simulink model "controller_test_lqg"  (R2015a)
settings: Solver=FixedStepDiscrete  StartTime=0.0  StopTime=40  FixedStep=0.02  RelTol=1e-3
values from neighbouring files (symbols this model uses):
  A = [2.32106176877 1 0 0 0 0 0 -0.677256428753 0 1 0 0 ... (49 elements, 7x7)]    [identified_sys_model.mat]
  B = [1 0 0 0 0 0 0]    [identified_sys_model.mat]
  C = [-0.0947664146756 0.174494212895 0 0 0 0 0]    [identified_sys_model.mat]
  M = iddata(yf2,u2detrended)    [model_identification_tests.m]
  Nbar = Nu+K*Nx    [controller_test.m]
undefined symbols (not defined in the file or in its folder): K
settings Model: ExtModeTrigDuration=200000  Creator=alunos  LastModifiedBy=jmgri
settings DataIOCC: LimitDataPoints=off
settings HardwareCC: ProdBitPerPointer=64  ProdLargestAtomicFloat=Float  ProdIntDivRoundTo=Zero  ProdEndianess=LittleEndian  ProdHWDeviceType=Specified  TargetIntDivRoundTo=Zero  TargetEndianess=LittleEndian  TargetHWDeviceType=Intel->x86/Pentium
settings RTWCC: SystemTargetFile=rtwin.tlc  TemplateMakefile=rtwin.tmf  Description=Simulink Desktop Real-Time  RTWCompilerOptimization=on
settings CodeAppCC: MaxIdLength=95
settings RTWinTargetCC: TargetPreCompLibLocation=C:\Program Files\MATLAB\R2017a\toolbox\sldrt\lib\win64  GeneratePreprocessorConditionals=Use local settings  ExtModeMexFile=sldrtext

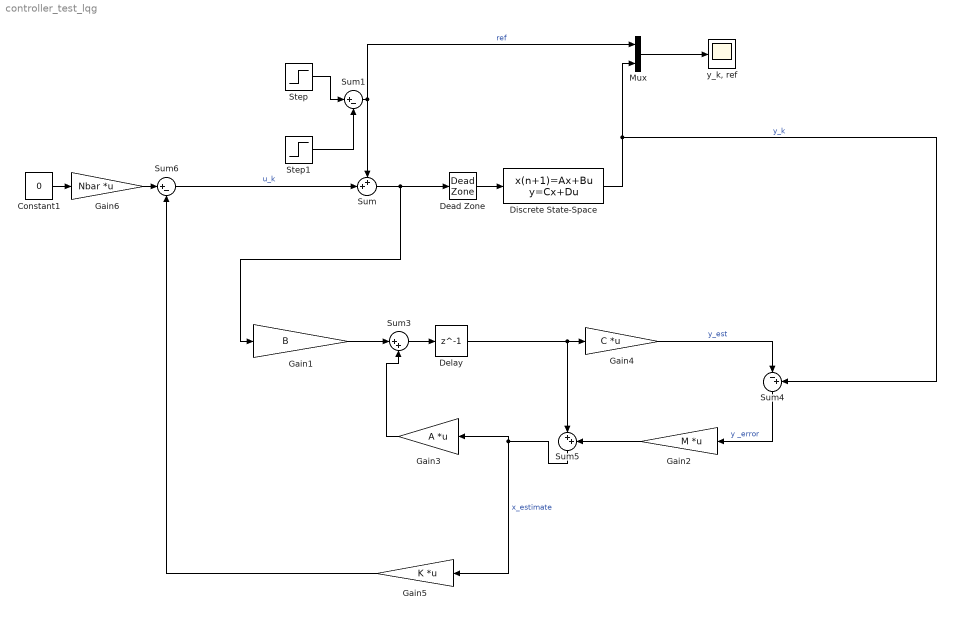
== system controller_test_lqg ==
  Constant1 : Constant  Value=0
  Dead Zone : DeadZone  LowerValue=-0.471  UpperValue=0.471  SaturateOnIntegerOverflow=on
  Delay : Delay  DelayLength=1
  Discrete State-Space : DiscreteStateSpace  A=A  B=B  C=[C]  D=[0]  SampleTime=-1
  Gain1 : Gain  Gain=B
  Gain2 : Gain  Gain=M  Multiplication=Matrix(K*u)
  Gain3 : Gain  Gain=A  Multiplication=Matrix(K*u)
  Gain4 : Gain  Gain=C  Multiplication=Matrix(K*u)
  Gain5 : Gain  Gain=K  Multiplication=Matrix(K*u)
  Gain6 : Gain  Gain=Nbar  Multiplication=Matrix(K*u)
  Mux : Mux  Inputs=2
  Step : Step
  Step1 : Step  Time=2
  Sum : Sum  Inputs=++|
  Sum1 : Sum  Inputs=|+-
  Sum3 : Sum  Inputs=|++
  Sum4 : Sum  Inputs=|-+
  Sum5 : Sum  Inputs=|++
  Sum6 : Sum  Inputs=|+-
  "y_k, ref" : Scope
      settings: TickLabels=on  SaveName=simulation_data  SampleInput=on
  wires:
  Mux/1 -> "y_k, ref"/1
  Step/1 -> Sum1/1
  Step1/1 -> Sum1/2
  Gain1/1 -> Sum3/1
  Sum3/1 -> Delay/1
  Delay/1 -> Gain4/1, Sum5/1
  Sum4/1 -> Gain2/1  "y _error"
  Gain2/1 -> Sum5/2
  Gain3/1 -> Sum3/2
  Discrete State-Space/1 -> Sum4/2, Mux/2  "y_k"
  Sum5/1 -> Gain3/1, Gain5/1  "x_estimate"
  Gain4/1 -> Sum4/1  "y_est"
  Sum/1 -> Dead Zone/1, Gain1/1
  Sum1/1 -> Sum/1, Mux/1  "ref"
  Sum6/1 -> Sum/2  "u_k"
  Gain5/1 -> Sum6/2
  Gain6/1 -> Sum6/1
  Constant1/1 -> Gain6/1
  Dead Zone/1 -> Discrete State-Space/1
